simulink model "s0506_rollsensorfusion_LKF"  (R2021a)
settings: Solver=FixedStepAuto  StartTime=0.0  StopTime=10.0  FixedStep=0.001  RelTol=1e-3
undefined symbols (not defined in the file or in its folder): Continuous, Time, X0
libraries: CarMaker4SL x28, ctrlSharedLib x1, cstblocks x1, simulink_extras x1
settings Model: Creator=jason  LastModifiedBy=jason

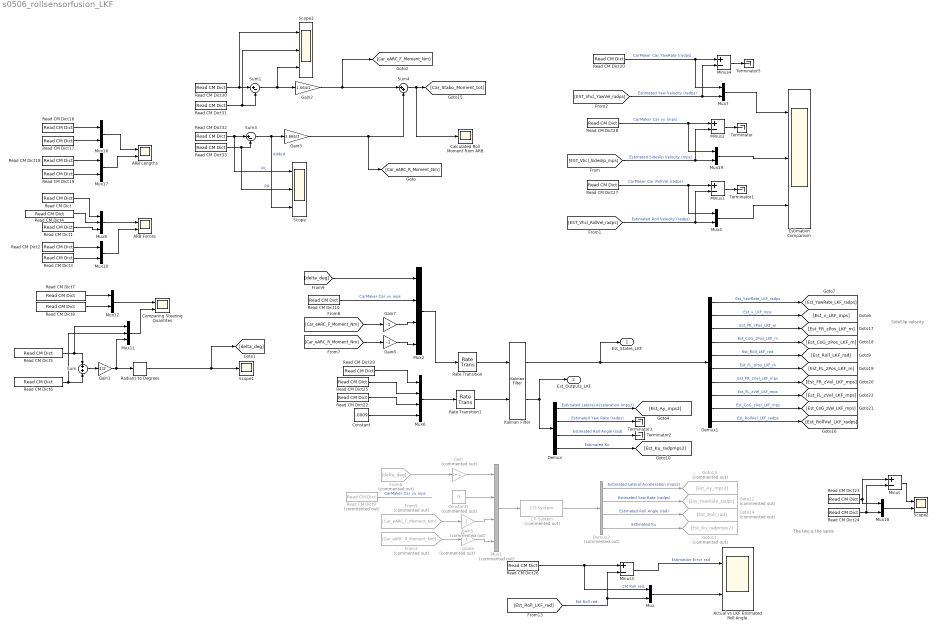
== system s0506_rollsensorfusion_LKF ==
  note: SideSlip velocity
  note: The two is the same
  ARB Forces : Scope  NumInputPorts=2
  ARB Lengths : Scope  NumInputPorts=2
  Actual vs LKF Estimated Roll Angle : Scope  NumInputPorts=2
  "Calculated Roll Moment from ARB " : Scope
  "Comparing Steering Quantites " : Scope  NumInputPorts=2
  Constant : Constant  Value=.0009
  Constant1 : Constant  Commented=on  Value=0
  Demux : Demux
      settings: DisplayOption=none
  Demux1 : Demux  Outputs=10
      settings: DisplayOption=none
  Demux2 : Demux  Commented=on
      settings: DisplayOption=none
  Estimation Comparison : Scope  NumInputPorts=3
  From3 : From  Commented=on  GotoTag=Car_eARC_R_Moment_Nm
  From5 : From  Commented=on  GotoTag=Car_eARC_F_Moment_Nm
  From6 : From  Commented=on  GotoTag=delta_deg
  Gain : Gain  Commented=on  Gain=1e-2
  Gain1 : Gain  Gain=1/2
  Gain2 : Gain  Gain=1.664/2
  Gain3 : Gain  Gain=1.665/2
  Gain5 : Gain  Commented=on  Gain=-1
  Gain6 : Gain  Commented=on  Gain=-1
  Gain7 : Gain  Gain=-1
  Gain8 : Gain  Gain=-1
  Goto11 : Goto  Commented=on  GotoTag=Est_Ku_radpmps2
  Goto12 : Goto  Commented=on  GotoTag=Est_YawRate_radps
  Goto13 : Goto  Commented=on  GotoTag=Est_Ay_mps2
  Goto14 : Goto  Commented=on  GotoTag=Est_Roll_rad
  Kalman Filter : ctrlSharedLib/Kalman Filter  TimeDomain=Continuous-Time  UseCurrentEstimator=on  ModelSource=LTI State-Space Variable  ModelSourceVariable=P_ss  A=0.95  B=1  C=1  D=0  NumberOfStates=1  NumberOfInputs=1  NumberOfOutputs=1  InitialEstimateSource=Dialog  X0=X0  P0=10  UseK=off  UseGH=off  NumberOfProcessNoiseInputs=1  G=1  TimeInvariantG=on  H=0  TimeInvariantH=on  Q=diag([0 0 0 0 0 0 0 0 0 0])  TimeInvariantQ=on  R=1  TimeInvariantR=on  N=0  TimeInvariantN=on  AddInputPort=on  AddEnablePort=off  OutputEstimatedY=on  OutputP=off  Ts=-1
  LTI System : cstblocks/LTI System  Commented=on  sys=P_ss  IC=[]
  Minus{,1..4} (5 alike) : Sum  Inputs=+-
  Mux{,4,7,10,12,16..19} (9 alike) : Mux  Inputs=2
  Mux1 : Mux  Commented=on
  Mux11 : Mux  Inputs=3
  Mux2 : Mux
  Mux6 : Mux
  Mux9 : Mux  Inputs=3
  Radians to Degrees : simulink_extras/Transformations/Radians to Degrees
  Rate Transition : RateTransition
  Rate Transition1 : RateTransition
  Read CM Dict : CarMaker4SL/Read CM Dict  xname=Car.StabiFL.Frc  xsync=off  xstime=Continuous
  Read CM Dict1 : CarMaker4SL/Read CM Dict  xname=Car.StabiFR.Frc  xsync=off  xstime=Continuous
  Read CM Dict10 : CarMaker4SL/Read CM Dict  xname=Car.vx  xsync=off  xstime=Continuous
  Read CM Dict16 : CarMaker4SL/Read CM Dict  xname=Car.StabiFL.l  xsync=off  xstime=Continuous
  Read CM Dict17 : CarMaker4SL/Read CM Dict  xname=Car.StabiFR.l  xsync=off  xstime=Continuous
  Read CM Dict18 : CarMaker4SL/Read CM Dict  xname=Car.StabiRL.l  xsync=off  xstime=Continuous
  Read CM Dict19 : CarMaker4SL/Read CM Dict  xname=Car.StabiRR.l  xsync=off  xstime=Continuous
  Read CM Dict2 : CarMaker4SL/Read CM Dict  xname=Car.StabiRL.Frc  xsync=off  xstime=Continuous
  Read CM Dict20 : CarMaker4SL/Read CM Dict  xname=Car.YawRate  xsync=off  xstime=Continuous
  Read CM Dict22 : CarMaker4SL/Read CM Dict  xname=Car.Roll  xsync=off  xstime=Continuous
  Read CM Dict23 : CarMaker4SL/Read CM Dict  xname=Car.YawRate  xsync=off  xstime=Continuous
  Read CM Dict24 : CarMaker4SL/Read CM Dict  xname=Car.YawVel  xsync=off  xstime=Continuous
  Read CM Dict25 : CarMaker4SL/Read CM Dict  xname=Car.YawRate  xsync=off  xstime=Continuous
  Read CM Dict26 : CarMaker4SL/Read CM Dict  xname=Car.Roll  xsync=off  xstime=Continuous
  Read CM Dict27 : CarMaker4SL/Read CM Dict  xname=Car.RollVel  xsync=off  xstime=Continuous
  Read CM Dict28 : CarMaker4SL/Read CM Dict  xname=Car.vy  xsync=off  xstime=Continuous
  Read CM Dict29 : CarMaker4SL/Read CM Dict  xname=Car.alHori  xsync=off  xstime=Continuous
  Read CM Dict3 : CarMaker4SL/Read CM Dict  xname=Car.StabiRR.Frc  xsync=off  xstime=Continuous
  Read CM Dict30 : CarMaker4SL/Read CM Dict  xname=Car.StabiFL.Frc  xsync=off  xstime=Continuous
  Read CM Dict31 : CarMaker4SL/Read CM Dict  xname=Car.StabiFR.Frc  xsync=off  xstime=Continuous
  Read CM Dict32 : CarMaker4SL/Read CM Dict  xname=Car.StabiRL.Frc  xsync=off  xstime=Continuous
  Read CM Dict33 : CarMaker4SL/Read CM Dict  xname=Car.StabiRR.Frc  xsync=off  xstime=Continuous
  Read CM Dict4 : CarMaker4SL/Read CM Dict  xname=Car.StabiFL.Frc_tot  xsync=off  xstime=Continuous
  Read CM Dict5 : CarMaker4SL/Read CM Dict  xname=Car.SteerAngleFL  xsync=off  xstime=Continuous
  Read CM Dict6 : CarMaker4SL/Read CM Dict  xname=Car.SteerAngleFR  xsync=off  xstime=Continuous
  Read CM Dict7 : CarMaker4SL/Read CM Dict  xname=Car.SteerAngleRL  xsync=off  xstime=Continuous
  Read CM Dict8 : CarMaker4SL/Read CM Dict  xname=Car.SteerAngleRR  xsync=off  xstime=Continuous
  Read CM Dict9 : CarMaker4SL/Read CM Dict  Commented=on  xname=Car.vx  xsync=off  xstime=Continuous
  Scope : Scope  NumInputPorts=3
  Scope1 : Scope
  Scope2 : Scope  NumInputPorts=2
  Scope3 : Scope  NumInputPorts=3
  Sum : Sum  Inputs=+|+
  Sum1 : Sum  Inputs=|+-
  Sum3 : Sum  Inputs=|+-
  Sum4 : Sum  Inputs=|++
  Terminator{,1..3,5} (5 alike) : Terminator
  Est_States_LKF : Outport
  Est_Outputs_LKF : Outport  Port=2
  wires:
  Minus4/1 -> Terminator5/1
  [EST_Vhcl_YawVel_radps] -> Minus4/2, Mux7/2  "Estimated Yaw Velocity (radps)"
  Mux19/1 -> Estimation Comparison/2
  Minus1/1 -> Terminator1/1
  Minus2/1 -> Terminator/1
  Mux4/1 -> Estimation Comparison/3
  Mux7/1 -> Estimation Comparison/1
  [EST_Vhcl_Sideslip_mps] -> Minus2/2, Mux19/2  "Estimated Sideslip Velocity (mps)"
  Demux/1 -> [Est_Ay_mps2]  "Estimated Lateral Acceleration (mps2)"
  Mux18/1 -> Scope2/2
  Read CM Dict27/1 -> Mux4/1, Minus1/1  "CarMaker Car.RollVel (radps)"
  Demux/2 -> Terminator3/1  "Estimated Yaw Rate (radps)"
  Read CM Dict28/1 -> Mux19/1, Minus2/1  "CarMaker Car.vy (mps)"
  Read CM Dict18/1 -> Mux17/1
  Read CM Dict16/1 -> Mux16/1
  Mux10/1 -> ARB Forces/2
  Read CM Dict23/1 -> Mux18/1, Minus/1
  Mux9/1 -> ARB Forces/1
  Read CM Dict1/1 -> Mux9/3
  Read CM Dict4/1 -> Mux9/2
  Read CM Dict2/1 -> Mux10/1
  Demux/4 -> [Est_Ku_radpmps2]  "Estimated Ku"
  Mux/1 -> Actual vs LKF Estimated Roll Angle/2
  Rate Transition/1 -> Kalman Filter/1
  Read CM Dict31/1 -> Scope3/2, Sum1/2
  Kalman Filter/2 -> Est_Outputs_LKF/1, Demux/1
  Read CM Dict17/1 -> Mux16/2
  Read CM Dict24/1 -> Minus/2, Mux18/2
  Mux17/1 -> ARB Lengths/2
  Read CM Dict/1 -> Mux9/1
  Rate Transition1/1 -> Kalman Filter/2
  Mux16/1 -> ARB Lengths/1
  Read CM Dict33/1 -> Scope/2, Sum3/2  "RR"
  Demux/3 -> Terminator2/1  "Estimated Roll Angle (rad)"
  [EST_Vhcl_RollVel_radps] -> Minus1/2, Mux4/2  "Estimated Roll Velocity (radps)"
  Read CM Dict26/1 -> Mux/1, Minus3/1  "CM Roll rad"
  Gain3/1 -> [Car_eARC_R_Moment_Nm], Sum4/2
  Read CM Dict30/1 -> Scope3/1, Sum1/1
  Gain2/1 -> [Car_eARC_F_Moment_Nm], Sum4/1
  Read CM Dict3/1 -> Mux10/2
  Mux6/1 -> Rate Transition1/1
  Minus/1 -> Scope2/1
  Read CM Dict19/1 -> Mux17/2
  Sum3/1 -> Scope/3, Gain3/1  "Added"
  Sum4/1 -> "Calculated Roll Moment from ARB "/1, [Car_Stabo_Moment_tot]
  Read CM Dict32/1 -> Scope/1, Sum3/1  "RL"
  Sum1/1 -> Scope3/3, Gain2/1
  Minus3/1 -> Actual vs LKF Estimated Roll Angle/1  "Estimation Error rad"
  Read CM Dict20/1 -> Mux7/1, Minus4/1  "CarMaker Car.YawRate (radps)"
  Read CM Dict5/1 -> Sum/1, Mux11/1
  Read CM Dict8/1 -> Mux12/2
  Sum/1 -> Gain1/1
  Gain1/1 -> Radians to Degrees/1, Mux11/3
  Mux11/1 -> "Comparing Steering Quantites "/2
  Read CM Dict6/1 -> Mux11/2, Sum/2
  Mux12/1 -> "Comparing Steering Quantites "/1
  Radians to Degrees/1 -> [delta_deg], Scope1/1
  Read CM Dict7/1 -> Mux12/1
  [Est_Roll_LKF_rad] -> Minus3/2, Mux/2  "Est Roll rad"
  Demux1/5 -> [Est_Roll_LKF_rad]  "Est_Roll_LKF_rad"
  Kalman Filter/1 -> Est_States_LKF/1, Demux1/1
  Demux1/2 -> [Est_v_LKF_mps]  "Est_v_LKF_mps"
  Demux1/1 -> [Est_YawRate_LKF_radps]  "Est_YawRate_LKF_radps"
  Mux1/1 -> LTI System/1
  Read CM Dict29/1 -> Mux6/1
  Read CM Dict25/1 -> Mux6/2
  Read CM Dict22/1 -> Mux6/3
  Constant/1 -> Mux6/4
  From5/1 -> Gain5/1
  Demux2/3 -> Goto14/1  "Estimated Roll Angle (rad)"
  Demux2/4 -> Goto11/1  "Estimated Ku"
  Demux2/1 -> Goto13/1  "Estimated Lateral Acceleration (mps2)"
  Demux2/2 -> Goto12/1  "Estimated Yaw Rate (radps)"
  LTI System/1 -> Demux2/1
  From3/1 -> Gain6/1
  Gain5/1 -> Mux1/3
  Gain6/1 -> Mux1/4
  From6/1 -> Gain/1
  Read CM Dict9/1 -> ?  "CarMaker Car.vx mps"
  Constant1/1 -> Mux1/2
  Gain/1 -> Mux1/1
  Gain7/1 -> Mux2/3
  Gain8/1 -> Mux2/4
  [Car_eARC_F_Moment_Nm] -> Gain7/1
  [delta_deg] -> Mux2/1
  [Car_eARC_R_Moment_Nm] -> Gain8/1
  Read CM Dict10/1 -> Mux2/2  "CarMaker Car.vx mps"
  Mux2/1 -> Rate Transition/1
  Demux1/10 -> [Est_RollVel_LKF_radps]  "Est_RollVel_LKF_radps"
  Demux1/3 -> [Est_FR_zPos_LKF_m]  "Est_FR_zPos_LKF_m"
  Demux1/4 -> [Est_CoG_zPos_LKF_m]  "Est_CoG_zPos_LKF_m"
  Demux1/6 -> [Est_FL_zPos_LKF_m]  "Est_FL_zPos_LKF_m"
  Demux1/7 -> [Est_FR_zVel_LKF_mps]  "Est_FR_zVel_LKF_mps"
  Demux1/9 -> [Est_CoG_zVel_LKF_mps]  "Est_CoG_zVel_LKF_mps"
  Demux1/8 -> [Est_FL_zVel_LKF_mps]  "Est_FL_zVel_LKF_mps"
